simulink model "FloatingPointIIR_DFormII"  (R2020a)
settings: Solver=VariableStepAuto  StartTime=0.0  StopTime=500  RelTol=1e-3
PreLoadFcn:
  | FloatingPointIIR_DFormII_PreLoadFcn
InitFcn:
  | xlIIRFilterResponse;
undefined symbols (not defined in the file): DEN2, DEN3, Fs, NUM1, NUM3, scale, xlIIRFilterResponse
libraries: xbsIndex_r4 x23, xbsCopyrightNotice_r4 x1
settings Model: Creator=viswanad  LastModifiedBy=viswanad
settings DataIOCC: ReturnWorkspaceOutputs=off
settings DebuggingCC: ArithmeticOperatorsInVariantConditions=warning
settings SFSimCC: SimUseLocalCustomCode=off  CustomCodeUndefinedFunction=UseInterfaceOnly
settings RTWCC: RTWUseLocalCustomCode=off
settings CodeAppCC: StateflowObjectComments=on

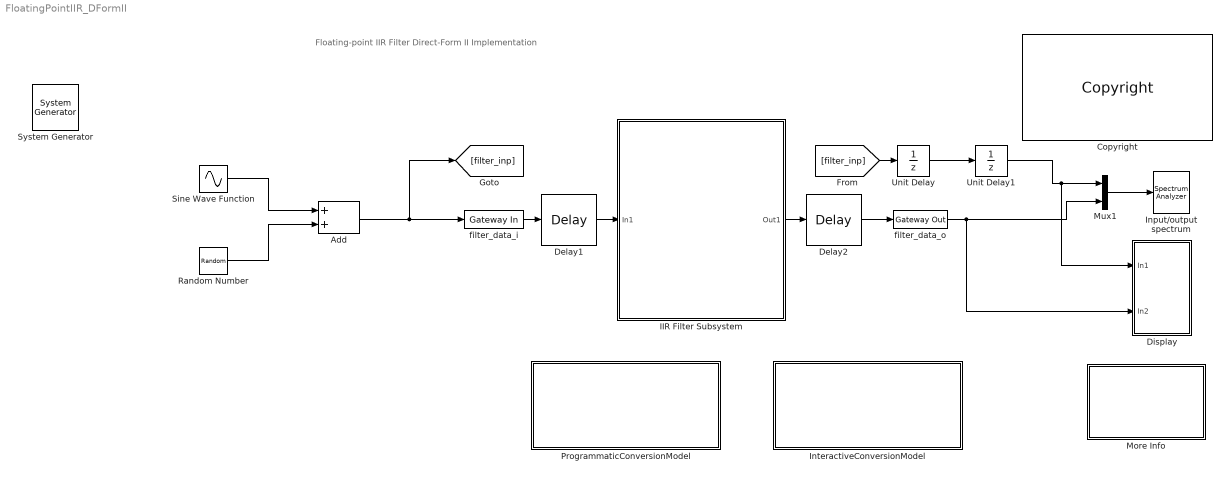
== system FloatingPointIIR_DFormII ==
  note: Floating-point IIR Filter Direct-Form II Implementation
  " System Generator" : xbsIndex_r4/ System Generator  Tag=genX  xilinxfamily=kintex7  part=xc7k325t  speed=-3  package=fbg676  synthesis_tool=Vivado  clock_wrapper=Clock Enables  directory=./netlist  proj_type=Vivado  Synth_file=Vivado Synthesis Defaults  Impl_file=Vivado Implementation Defaults  testbench=off  simulink_period=1/(scale*Fs)  sysclk_period=10  dcm_input_clock_period=10  incr_netlist=off  trim_vbits=Everywhere in SubSystem  dbl_ovrd=According to Block Masks  core_generation=According to Block Masks  run_coregen=off  deprecated_control=off  eval_field=0  block_type=sysgen
  Add : Sum
  Copyright : xbsCopyrightNotice_r4/Copyright  copyrighttext="Copyright (c) 2021  by  Xilinx, Inc. All rights reserved.<br><br>This file contains proprietary, confidential information of Xilinx, Inc., is distributed under license from Xilinx, Inc., and may be used, copied and/or disclosed only pursuant to the terms of a valid license agreement with Xilinx, Inc. Xilinx hereby grants you a license to use this file solely for design, simulation, implementation and creation of design files limited to Xilinx devices or technologies. Use with non-Xilinx devices or technologies is expressly prohibited and immediately terminates your license unless covered by a separate agreement.<br><br>Xilinx is providing this design, code, or information \"as-is\" solely for use in developing programs and solutions for Xilinx devices, with no obligation on the part of Xilinx to provide support. By providing this design, code, or information as one possible implementation of this feature, application or standard, Xilinx is making no representation that this implementation is free from any claims of infringement. You are responsible for obtaining any rights you may require for your implementation. Xilinx expressly disclaims any warranty whatsoever with respect to the adequacy of the implementation, including but not limited to any warranties or representations that this implementation is free from claims of infringement, implied warranties of merchantability or fitness for a particular purpose.<br><br>Xilinx products are not intended for use in life support appliances, devices, or systems. Use in such applications is expressly prohibited.<br><br>Any modifications that are made to the Source Code are done at the user's sole risk and will be unsupported.<br><br>This copyright and support notice must be retained as part of this text at all times. (c) Copyright 1995-2021 Xilinx, Inc. All rights reserved."  block_type=copyright
  Delay1 : xbsIndex_r4/Delay  rst=off  en=off  latency=1  reg_retiming=off  XmcBlockStatus=1  maskContainerNames=group1  block_type=delay  block_config=sysgen:Delay_config
  Delay2 : xbsIndex_r4/Delay  rst=off  en=off  latency=1  reg_retiming=off  XmcBlockStatus=1  maskContainerNames=group1  block_type=delay  block_config=sysgen:Delay_config
  Display : Subsystem
  IIR Filter Subsystem : Subsystem
  Input/output spectrum : SpectrumAnalyzer
  InteractiveConversionModel : Subsystem
      settings: OpenFcn=xlConvertModel_I();
      mask Display: disp('Double click\n  to\n  switch between\n  Fixed-point and Floating-point\n  interactively');
  More Info : Subsystem
      mask Display: disp('Double click\n for\n more information.')
  Mux1 : Mux  Inputs=2
  ProgrammaticConversionModel : Subsystem
      settings: OpenFcn=xlConvertModel_P();
      mask Display: disp('Double click\n  to\n  switch between\n  Fixed-point and Floating-point\n  programmatically');
  Random Number : RandomNumber  Variance=10  SampleTime=1/(Fs)
  Sine Wave Function : Sin  Frequency=2*3.14*5000  SampleTime=1/(Fs)
  Unit Delay : UnitDelay  SampleTime=-1  HasFrameUpgradeWarning=on
  Unit Delay1 : UnitDelay  SampleTime=-1  HasFrameUpgradeWarning=on
  filter_data_i : xbsIndex_r4/Gateway In  gui_display_data_type=Floating-point  arith_type=Floating-point  n_bits=32  bin_pt=24  preci_type=Custom  exp_width=6  frac_width=9  rows=1  columns=1  quantization="Round  (unbiased: +/- Inf)"  overflow=Saturate  period=1/(Fs)  UseAsADC=off  ADCChannel='1'  interface=None  automatic_assignment=on  address_offset=hex2dec('00')  intf_name=''  intf_description=''  default_value=0  timing_constraint=None  locs_specified=off  LOCs={}  io_standard={}  inherit_from_input=off  hdl_port=on  XmcBlockStatus=1  maskContainerNames=group4  block_type=gatewayin  block_config=sysgen:gateway_in_config
  filter_data_o : xbsIndex_r4/Gateway Out  inherit_from_input=off  hdl_port=on  rows=1  columns=1  UseAsDAC=off  DACChannel='1'  interface=None  automatic_assignment=on  address_offset=hex2dec('00')  intf_name=''  intf_description=''  timing_constraint=None  locs_specified=off  LOCs={}  io_standard={}  XmcBlockStatus=1  maskContainerNames=group4  block_type=gatewayout  block_config=sysgen:gateway_out_config
  wires:
  Delay1/1 -> IIR Filter Subsystem/1(In1)
  filter_data_i/1 -> Delay1/1
  Add/1 -> filter_data_i/1, [filter_inp]
  filter_data_o/1 -> Mux1/2, Display/2(In2)
  Random Number/1 -> Add/2
  Unit Delay/1 -> Unit Delay1/1
  IIR Filter Subsystem/1(Out1) -> Delay2/1
  Delay2/1 -> filter_data_o/1
  Sine Wave Function/1 -> Add/1
  Mux1/1 -> Input/output spectrum/1
  Unit Delay1/1 -> Mux1/1, Display/1(In1)
  [filter_inp] -> Unit Delay/1

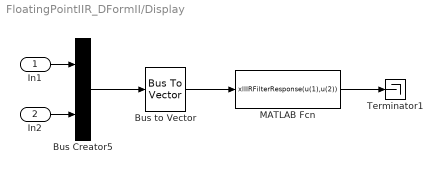
== system FloatingPointIIR_DFormII/Display ==
  In1 : Inport
  In2 : Inport  Port=2
  Bus Creator5 : BusCreator  Inputs=2
  Bus to Vector : BusToVector
  MATLAB Fcn : MATLABFcn  MATLABFcn=xlIIRFilterResponse(u(1),u(2))
  Terminator1 : Terminator
  wires:
  MATLAB Fcn/1 -> Terminator1/1
  Bus to Vector/1 -> MATLAB Fcn/1
  Bus Creator5/1 -> Bus to Vector/1
  In1/1 -> Bus Creator5/1
  In2/1 -> Bus Creator5/2

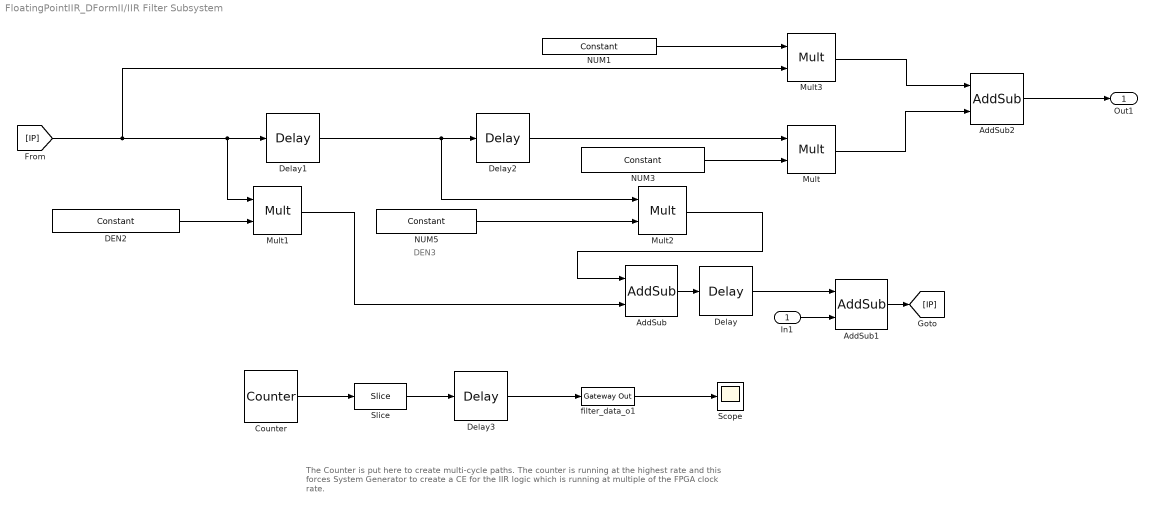
== system FloatingPointIIR_DFormII/IIR Filter Subsystem ==
  note: DEN3
  note: The Counter is put here to create multi-cycle paths. The counter is running at the highest rate
      | and this forces System Generator  to create a CE for the IIR logic which is running at multiple of  the
      | FPGA clock rate.
  In1 : Inport
  AddSub : xbsIndex_r4/AddSub  mode=Addition  use_carryin=off  use_carryout=off  en=off  latency=0  precision=Full  arith_type="Signed  (2's comp)"  n_bits=32  bin_pt=24  quantization=Truncate  overflow=Wrap  use_behavioral_HDL=off  hw_selection=DSP48  pipelined=off  XmcBlockStatus=1  maskContainerNames=tabcontainer1  block_type=addsub  block_config=sysgen:Addsub_config
  AddSub1 : xbsIndex_r4/AddSub  mode=Addition  use_carryin=off  use_carryout=off  en=off  latency=0  precision=Full  arith_type="Signed  (2's comp)"  n_bits=32  bin_pt=24  quantization=Truncate  overflow=Wrap  use_behavioral_HDL=off  hw_selection=DSP48  pipelined=off  XmcBlockStatus=1  maskContainerNames=tabcontainer1  block_type=addsub  block_config=sysgen:Addsub_config
  AddSub2 : xbsIndex_r4/AddSub  mode=Addition  use_carryin=off  use_carryout=off  en=off  latency=0  precision=Full  arith_type="Signed  (2's comp)"  n_bits=32  bin_pt=24  quantization=Truncate  overflow=Wrap  use_behavioral_HDL=off  hw_selection=DSP48  pipelined=off  XmcBlockStatus=1  maskContainerNames=tabcontainer1  block_type=addsub  block_config=sysgen:Addsub_config
  Counter : xbsIndex_r4/Counter  cnt_type=Free Running  cnt_to=Inf  operation=Up  start_count=0  cnt_by_val=1  arith_type=Unsigned  n_bits=4  bin_pt=0  load_pin=off  rst=off  en=off  explicit_period=on  period=1/(scale*Fs)  use_behavioral_HDL=off  implementation=Fabric  XmcBlockStatus=1  maskContainerNames=group1  block_type=counter  block_config=sysgen:Counter_config
  DEN2 : xbsIndex_r4/Constant  const=DEN2  gui_display_data_type=Floating-point  arith_type=Floating-point  n_bits=32  bin_pt=24  preci_type=Custom  exp_width=6  frac_width=9  explicit_period=on  period=1/(Fs)  XmcBlockStatus=1  maskContainerNames=tabcontainer1  block_type=constant  block_config=sysgen:Constant_config
  Delay{,1..3} (4 alike) : xbsIndex_r4/Delay  rst=off  en=off  latency=1  reg_retiming=off  XmcBlockStatus=1  maskContainerNames=group1  block_type=delay  block_config=sysgen:Delay_config
  Mult{,1..3} (4 alike) : xbsIndex_r4/Mult  precision=Full  arith_type="Signed  (2's comp)"  n_bits=32  bin_pt=24  quantization=Truncate  overflow=Wrap  en=off  latency=0  use_behavioral_HDL=off  opt=Speed  use_embedded=on  optimum_pipeline=off  pipeline=on  use_rpm=on  placement_style=Triangular  XmcBlockStatus=1  maskContainerNames=group1  block_type=mult  block_config=sysgen:Mult_config
  NUM1 : xbsIndex_r4/Constant  const=NUM1  gui_display_data_type=Floating-point  arith_type=Floating-point  n_bits=32  bin_pt=24  preci_type=Custom  exp_width=6  frac_width=9  explicit_period=on  period=1/(Fs)  XmcBlockStatus=1  maskContainerNames=tabcontainer1  block_type=constant  block_config=sysgen:Constant_config
  NUM3 : xbsIndex_r4/Constant  const=NUM3  gui_display_data_type=Floating-point  arith_type=Floating-point  n_bits=32  bin_pt=24  preci_type=Custom  exp_width=6  frac_width=9  explicit_period=on  period=1/(Fs)  XmcBlockStatus=1  maskContainerNames=tabcontainer1  block_type=constant  block_config=sysgen:Constant_config
  NUM5 : xbsIndex_r4/Constant  const=DEN3  gui_display_data_type=Floating-point  arith_type=Floating-point  n_bits=32  bin_pt=24  preci_type=Custom  exp_width=6  frac_width=9  explicit_period=on  period=1/(Fs)  XmcBlockStatus=1  maskContainerNames=tabcontainer1  block_type=constant  block_config=sysgen:Constant_config
  Scope : Scope
  Slice : xbsIndex_r4/Slice  nbits=4  boolean_output=off  mode=Upper Bit Location + Width  bit1=0  base1=MSB of Input  bit0=0  base0=LSB of Input  XmcBlockStatus=1  maskContainerNames=group1  block_type=slice  block_config=sysgen:Slice_config
  filter_data_o1 : xbsIndex_r4/Gateway Out  inherit_from_input=off  hdl_port=off  rows=1  columns=1  UseAsDAC=off  DACChannel='1'  interface=None  automatic_assignment=on  address_offset=hex2dec('00')  intf_name=''  intf_description=''  timing_constraint=None  locs_specified=off  LOCs={}  io_standard={}  XmcBlockStatus=1  maskContainerNames=group4  block_type=gatewayout  block_config=sysgen:gateway_out_config
  Out1 : Outport  VectorParamsAs1DForOutWhenUnconnected=off
  wires:
  Delay1/1 -> Mult2/1, Delay2/1
  NUM3/1 -> Mult/2
  DEN2/1 -> Mult1/2
  NUM5/1 -> Mult2/2
  Mult1/1 -> AddSub/2
  Mult2/1 -> AddSub/1
  NUM1/1 -> Mult3/1
  Mult3/1 -> AddSub2/1
  Mult/1 -> AddSub2/2
  [IP] -> Mult3/2, Delay1/1, Mult1/1
  AddSub2/1 -> Out1/1
  AddSub1/1 -> [IP]
  AddSub/1 -> Delay/1
  In1/1 -> AddSub1/2
  Delay/1 -> AddSub1/1
  Delay2/1 -> Mult/1
  Counter/1 -> Slice/1
  filter_data_o1/1 -> Scope/1
  Slice/1 -> Delay3/1
  Delay3/1 -> filter_data_o1/1

== system FloatingPointIIR_DFormII/InteractiveConversionModel ==

== system FloatingPointIIR_DFormII/More Info ==
  note: Floating-point IIR Filter Direct-Form II Implementation
  note: This design is a model for Direct Form II realization of a second-order IIR Filter (Peaking Filter).
      |
      | The design shows Sysgen's capability to switch between Floating point and Fixed point data.
      |
      | The same design can be modified to a Fixed-point model -
      |         a) Programmatically, using the 'ConversionModel' switch present at the top-level or
      |         b) Manually, by configuring different blocks in the system (a brief description available at the top-level)
      |
      | It can be noticed from the plotted filter-reponses, using a Floating-point system (Custom precision, Exponent-width=6, Fraction-width=9) it
      | achieves a  much better filter-response with less-than-half the total-bitwidth, when compared to the Fixed-point model (Number of bits = 32,
      | Binary point = 24).
      |
      | Implementation notes:
      |
      | For Floating-point system:
      | - Input precision ('Arithmetic type', 'Number of bits' and 'Binary point') at the GatewayIn and Constant block-GUIs should be same.
      | - Output precision at the Addsub and Multiplier blocks should be selected as 'Full' precision.
      |
      | For Fixed-point system:
      | -  Output precision ('Output type', 'Number of bits' and 'Binary point') at the Addsub and Multiplier block-GUIs should be specified explicitly,
      |     by selecting 'User defined' precision.
      |
      | The operating clock frequency for the top-level design as shown is 48KHz and input signal-frequency is 5KHz and SNR being ~ -13dB.
      |
      | At the top-level system, a counter is added to create multi-cycle paths. The counter is running at the highest rate and this forces
      | System Generator to create a CE for the IIR logic which is running at a multiple of  the FPGA clock rate.

== system FloatingPointIIR_DFormII/ProgrammaticConversionModel ==
